simulink model "gtrackpol15"  (R2017a)
settings: Solver=ode45  StartTime=0.0  StopTime=15  FixedStep=.1  RelTol=1e-3
libraries: simulink x2
settings Model: Creator=Dell  LastModifiedBy=Dell
settings OptimizationCC: LifeSpan=inf
settings DebuggingCC: SFExecutionAtInitializationDiag=none
settings HardwareCC: ProdBitPerSizeT=32  ProdBitPerPtrDiffT=32  ProdWordSize=32  ProdHWDeviceType=Specified

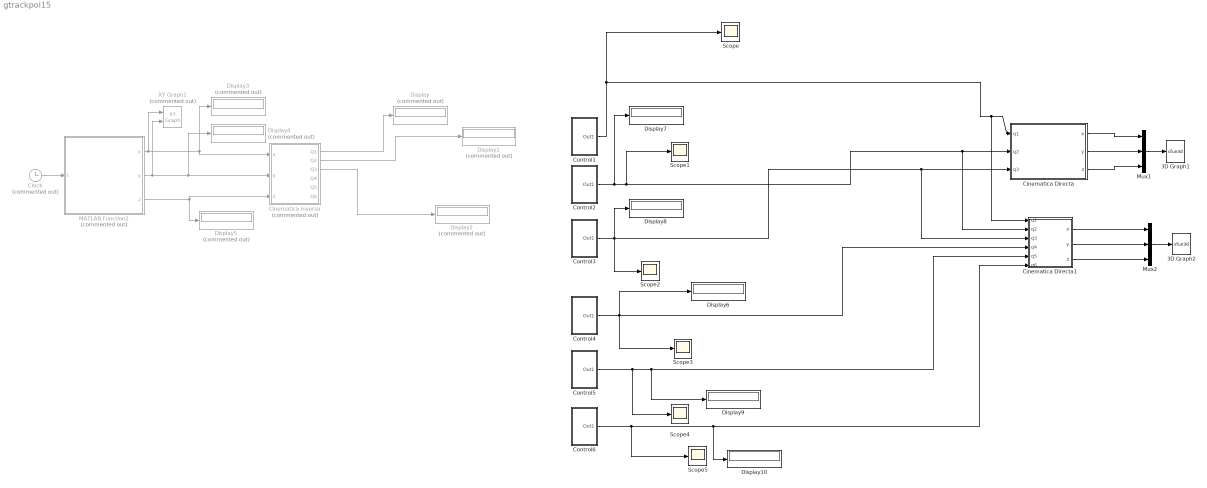
== system gtrackpol15 ==
  3D Graph1 : S-Function  LoadFcn=if exist('sfun3d','file'), sfun3d([],[],[],'LoadBlock'); end  FunctionName=sfun3d  Parameters=ax,T,np,cp,gd,ls,mk,mx,hd,tb  SFunctionDeploymentMode=off  EnableBusSupport=off  mask(3D Graph){np=1, ax=[-.7 0.7 -.7 0.7 -.7 .7], mx=2000, T=-1, cp=[370 -234 -207], gd=on, hd=on, tb=off, ls=-, mk=none}
      mask prompts: np "Number of moving points (lines)"; ax "Range: [xmin xmax  ymin ymax zmin zmax]"; mx "Max number of points in each line"; T "Sampling Time"; cp "Camera position (use [0 0 1] for 2D XY view)"; gd "Grid (on|off)"; hd "HeadMarkers (on|off)"; tb "Toolbar (on|off)"; ls "LineStyle"; mk "LineMarker"
      mask help:
      | This block plots the position of several points in the XYZ space. The input contains the coordinates of all the points (x1,y1,z1,x2,y2,z2,...).
      | The number of moving points (lines), the XYZ ranges, sampling time, camera position, and grid (among other things) can be set as mask parameters.
      settings: CopyFcn=if exist('sfun3d','file'), sfun3d([],[],[],'CopyBlock'); end  DeleteFcn=if exist('sfun3d','file'), sfun3d([],[],[],'DeleteBlock'); end  NameChangeFcn=if exist('sfun3d','file'), sfun3d([],[],[],'NameChange'); end
      mask Help:
      | This block plots the position of several points in the XYZ space. The input contains the coordinates of all the points (x1,y1,z1,x2,y2,z2,...).
      | The number of moving points (lines), the XYZ ranges, sampling time, camera position, and grid (among other things) can be set as mask parameters.
      mask TypeOptions ls: - | -- | : | -. | none
      mask TypeOptions mk: none | . | + | o | * | x | square | diamond | v | ^ | > | < | pentagram | hexagram
      mask Display: plot([.05 .95 .95 .05 .05],[.45 .45 .95 .95 .45], 0.5+cos(0:0.1:2*pi)*0.3,0.7+sin(0:0.1:2*pi)*0.2)
  3D Graph2 : S-Function  LoadFcn=if exist('sfun3d','file'), sfun3d([],[],[],'LoadBlock'); end  FunctionName=sfun3d  Parameters=ax,T,np,cp,gd,ls,mk,mx,hd,tb  SFunctionDeploymentMode=off  EnableBusSupport=off  mask(3D Graph){np=1, ax=[-.7 0.7 -.7 0.7 -.7 .7], mx=2000, T=-1, cp=[370 -234 -207], gd=on, hd=on, tb=off, ls=-, mk=none}
      mask prompts: np "Number of moving points (lines)"; ax "Range: [xmin xmax  ymin ymax zmin zmax]"; mx "Max number of points in each line"; T "Sampling Time"; cp "Camera position (use [0 0 1] for 2D XY view)"; gd "Grid (on|off)"; hd "HeadMarkers (on|off)"; tb "Toolbar (on|off)"; ls "LineStyle"; mk "LineMarker"
      mask help:
      | This block plots the position of several points in the XYZ space. The input contains the coordinates of all the points (x1,y1,z1,x2,y2,z2,...).
      | The number of moving points (lines), the XYZ ranges, sampling time, camera position, and grid (among other things) can be set as mask parameters.
      settings: CopyFcn=if exist('sfun3d','file'), sfun3d([],[],[],'CopyBlock'); end  DeleteFcn=if exist('sfun3d','file'), sfun3d([],[],[],'DeleteBlock'); end  NameChangeFcn=if exist('sfun3d','file'), sfun3d([],[],[],'NameChange'); end
      mask Help:
      | This block plots the position of several points in the XYZ space. The input contains the coordinates of all the points (x1,y1,z1,x2,y2,z2,...).
      | The number of moving points (lines), the XYZ ranges, sampling time, camera position, and grid (among other things) can be set as mask parameters.
      mask TypeOptions ls: - | -- | : | -. | none
      mask TypeOptions mk: none | . | + | o | * | x | square | diamond | v | ^ | > | < | pentagram | hexagram
      mask Display: plot([.05 .95 .95 .05 .05],[.45 .45 .95 .95 .45], 0.5+cos(0:0.1:2*pi)*0.3,0.7+sin(0:0.1:2*pi)*0.2)
  Cinematica Directa : MATLAB Function  TreatAsAtomicUnit=on
  Cinematica Directa1 : MATLAB Function  TreatAsAtomicUnit=on
  "Cinematica Inversa " : MATLAB Function  Commented=on  TreatAsAtomicUnit=on
  Clock : Clock  Commented=on
  "Control1 " : Subsystem
  Control2 : Subsystem
  "Control3 " : Subsystem
  "Control4 " : Subsystem
  Control5 : Subsystem
  Control6 : Subsystem
  Display{,1..5} (6 alike) : Display  Commented=on
  Display{6..10} (5 alike) : Display
  MATLAB Function2 : MATLAB Function  Commented=on  TreatAsAtomicUnit=on
  Mux1 : Mux  Inputs=3
  Mux2 : Mux  Inputs=3
  Scope{,1..5} (6 alike) : Scope
  XY Graph1 : simulink/Sinks/XY Graph  Commented=on  xmin=-1  xmax=1  ymin=-1  ymax=1  st=0.01
  wires:
  Control2/1(Out1) -> Cinematica Directa1/2(q2), Cinematica Directa/2(q2), Scope1/1, Display7/1
  MATLAB Function2/1(x) -> "Cinematica Inversa "/1(x), Display3/1, XY Graph1/1
  MATLAB Function2/3(z) -> "Cinematica Inversa "/3(z), Display5/1
  "Control1 "/1(Out1) -> Cinematica Directa1/1(q1), Cinematica Directa/1(q1), Scope/1
  "Cinematica Inversa "/3(Q3) -> Display2/1
  MATLAB Function2/2(y) -> XY Graph1/2, "Cinematica Inversa "/2(y), Display4/1
  "Cinematica Inversa "/2(Q2) -> Display1/1
  Clock/1 -> MATLAB Function2/1(t)
  "Cinematica Inversa "/1(Q1) -> Display/1
  Cinematica Directa/2(y) -> Mux1/2
  Cinematica Directa/3(z) -> Mux1/3
  Mux1/1 -> 3D Graph1/1
  Cinematica Directa/1(x) -> Mux1/1
  "Control3 "/1(Out1) -> Cinematica Directa1/3(q3), Cinematica Directa/3(q3), Scope2/1, Display8/1
  "Control4 "/1(Out1) -> Scope3/1, Display6/1, Cinematica Directa1/4(q4)
  Control5/1(Out1) -> Scope4/1, Display9/1, Cinematica Directa1/5(q5)
  Control6/1(Out1) -> Scope5/1, Display10/1, Cinematica Directa1/6(q6)
  Cinematica Directa1/1(x) -> Mux2/1
  Mux2/1 -> 3D Graph2/1
  Cinematica Directa1/3(z) -> Mux2/3
  Cinematica Directa1/2(y) -> Mux2/2

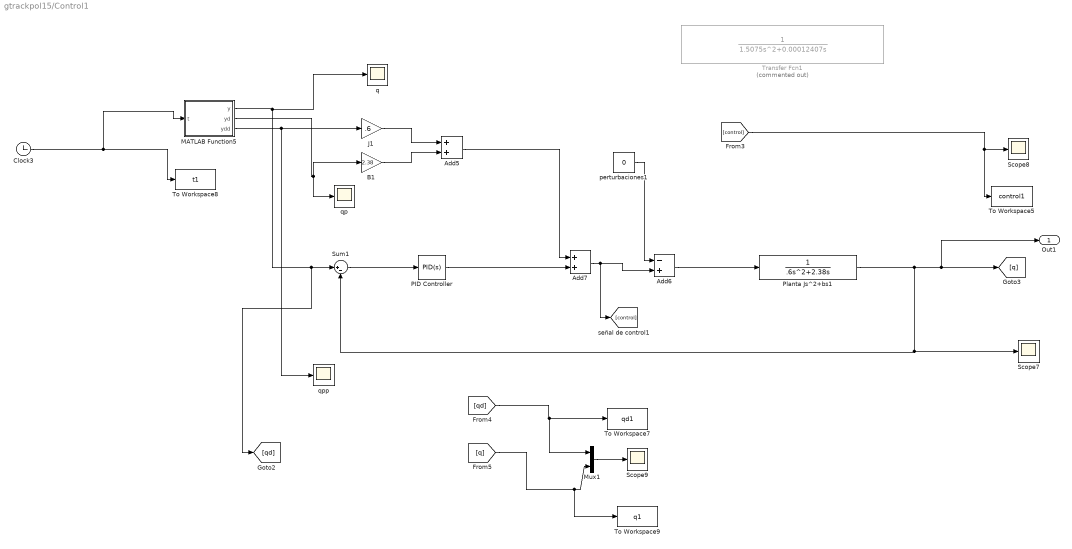
== system gtrackpol15/Control1  ==
  Add5 : Sum
  Add6 : Sum  Inputs=-+
  Add7 : Sum
  B1 : Gain  Gain=2.38
  Clock3 : Clock
  J1 : Gain  Gain=.6
  MATLAB Function5 : MATLAB Function  TreatAsAtomicUnit=on
  Mux1 : Mux  Inputs=2
  PID Controller : simulink/Continuous/PID Controller  Controller=PID  TimeDomain=Continuous-time  SampleTime=-1  IntegratorMethod=Forward Euler  FilterMethod=Forward Euler  Form=Parallel  UseFilter=on  ControllerParametersSource=internal  P=10  I=0  D=1  N=1279.60012976235  InitialConditionSource=internal  InitialConditionForIntegrator=0  InitialConditionForFilter=0  ExternalReset=none  LimitOutput=on  UpperSaturationLimit=255  LowerSaturationLimit=-255  LinearizeAsGain=on  AntiWindupMode=none  Kb=1  TrackingMode=off  Kt=1  PParamMin=[]  PParamMax=[]  IParamMin=[]  IParamMax=[]  DParamMin=[]  DParamMax=[]  NParamMin=[]  NParamMax=[]  KbParamMin=[]  KbParamMax=[]  KtParamMin=[]  KtParamMax=[]  POutMin=[]  POutMax=[]  IOutMin=[]  IOutMax=[]  DOutMin=[]  DOutMax=[]  NOutMin=[]  NOutMax=[]  KbOutMin=[]  KbOutMax=[]  KtOutMin=[]  KtOutMax=[]  IntegratorOutMin=[]  IntegratorOutMax=[]  FilterOutMin=[]  FilterOutMax=[]  SumOutMin=[]  SumOutMax=[]  SumI1OutMin=[]  SumI1OutMax=[]  SumI2OutMin=[]  SumI2OutMax=[]  SumI3OutMin=[]  SumI3OutMax=[]  SumDOutMin=[]  SumDOutMax=[]  SaturationOutMin=[]  SaturationOutMax=[]  IntegratorContinuousStateAttributes=''  IntegratorStateMustResolveToSignalObject=off  IntegratorRTWStateStorageClass=Auto  FilterContinuousStateAttributes=''  FilterStateMustResolveToSignalObject=off  FilterRTWStateStorageClass=Auto  DifferentiatorICPrevScaledInput=0  DifferentiatorOutMin=[]  DifferentiatorOutMax=[]  InitialConditionSetting=State (most efficient)
  Planta Js^2+bs1 : TransferFcn  Denominator=[.6 2.38 0]
  Scope7 : Scope
  Scope8 : Scope
  Scope9 : Scope
  Sum1 : Sum  Inputs=|+-
  To Workspace5 : ToWorkspace  VariableName=control1  SampleTime=-1
  To Workspace7 : ToWorkspace  VariableName=qd1  SampleTime=-1
  To Workspace8 : ToWorkspace  VariableName=t1  SampleTime=-1
  To Workspace9 : ToWorkspace  VariableName=q1  SampleTime=-1
  Transfer Fcn1 : TransferFcn  Commented=on  Denominator=[1.5075 0.00012407 0]
  perturbaciones1 : Constant  Value=0
  q : Scope
  qp : Scope
  qpp : Scope
  Out1 : Outport
  wires:
  MATLAB Function5/2(yd) -> B1/1, qp/1
  Mux1/1 -> Scope9/1
  Sum1/1 -> PID Controller/1
  J1/1 -> Add5/1
  Add7/1 -> Add6/2, [control]
  PID Controller/1 -> Add7/2
  [control] -> Scope8/1, To Workspace5/1
  [q] -> Mux1/2, To Workspace9/1
  [qd] -> Mux1/1, To Workspace7/1
  Add5/1 -> Add7/1
  Clock3/1 -> To Workspace8/1, MATLAB Function5/1(t)
  MATLAB Function5/1(y) -> q/1, Sum1/1, [qd]
  B1/1 -> Add5/2
  perturbaciones1/1 -> Add6/1
  MATLAB Function5/3(ydd) -> qpp/1, J1/1
  Add6/1 -> Planta Js^2+bs1/1
  Planta Js^2+bs1/1 -> Sum1/2, Scope7/1, Out1/1, [q]

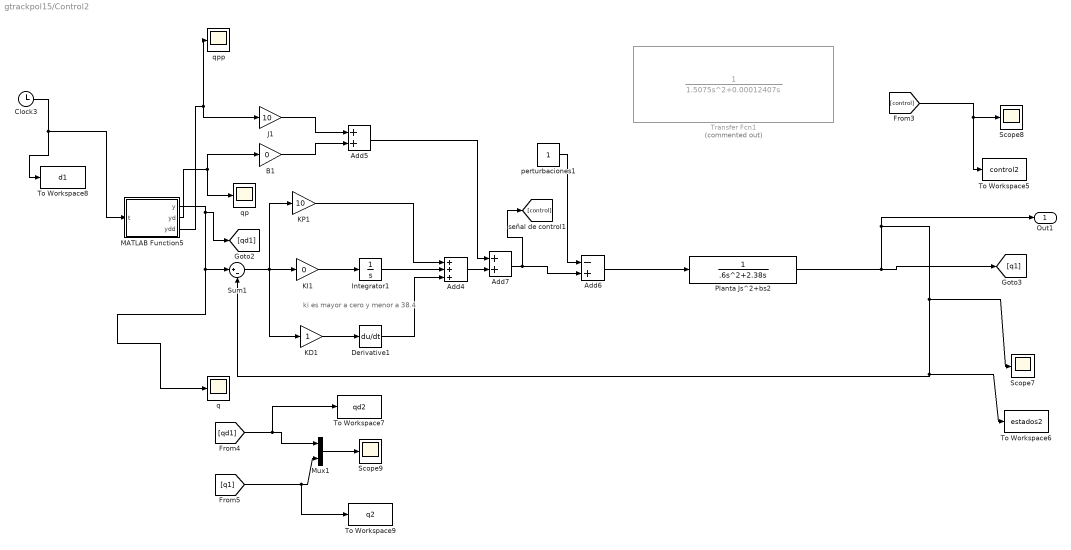
== system gtrackpol15/Control2 ==
  note: ki es mayor a cero y menor a 38.4
  Add4 : Sum  Inputs=+++
  Add5 : Sum
  Add6 : Sum  Inputs=-+
  Add7 : Sum
  B1 : Gain  Gain=0
  Clock3 : Clock
  Derivative1 : Derivative
  Integrator1 : Integrator
  J1 : Gain  Gain=10
  KD1 : Gain
  KI1 : Gain  Gain=0
  KP1 : Gain  Gain=10
  MATLAB Function5 : MATLAB Function  TreatAsAtomicUnit=on
  Mux1 : Mux  Inputs=2
  Planta Js^2+bs2 : TransferFcn  Denominator=[.6 2.38 0]
  Scope7 : Scope
  Scope8 : Scope
  Scope9 : Scope
  Sum1 : Sum  Inputs=|+-
  To Workspace5 : ToWorkspace  VariableName=control2  SampleTime=-1
  To Workspace6 : ToWorkspace  VariableName=estados2  SampleTime=-1
  To Workspace7 : ToWorkspace  VariableName=qd2  SampleTime=-1
  To Workspace8 : ToWorkspace  VariableName=d1  SampleTime=-1
  To Workspace9 : ToWorkspace  VariableName=q2  SampleTime=-1
  Transfer Fcn1 : TransferFcn  Commented=on  Denominator=[1.5075 0.00012407 0]
  perturbaciones1 : Constant
  q : Scope
  qp : Scope
  qpp : Scope
  Out1 : Outport
  wires:
  Derivative1/1 -> Add4/3
  perturbaciones1/1 -> Add6/1
  B1/1 -> Add5/2
  MATLAB Function5/1(y) -> [qd1], q/1, Sum1/1
  KD1/1 -> Derivative1/1
  Add5/1 -> Add7/1
  Integrator1/1 -> Add4/2
  MATLAB Function5/3(ydd) -> qpp/1, J1/1
  [qd1] -> To Workspace7/1, Mux1/1
  [q1] -> To Workspace9/1, Mux1/2
  KI1/1 -> Integrator1/1
  [control] -> To Workspace5/1, Scope8/1
  Add4/1 -> Add7/2
  Add7/1 -> [control], Add6/2
  J1/1 -> Add5/1
  Sum1/1 -> KD1/1, KI1/1, KP1/1
  Mux1/1 -> Scope9/1
  KP1/1 -> Add4/1
  MATLAB Function5/2(yd) -> qp/1, B1/1
  Add6/1 -> Planta Js^2+bs2/1
  Planta Js^2+bs2/1 -> Scope7/1, To Workspace6/1, Sum1/2, Out1/1, [q1]
  Clock3/1 -> MATLAB Function5/1(t), To Workspace8/1

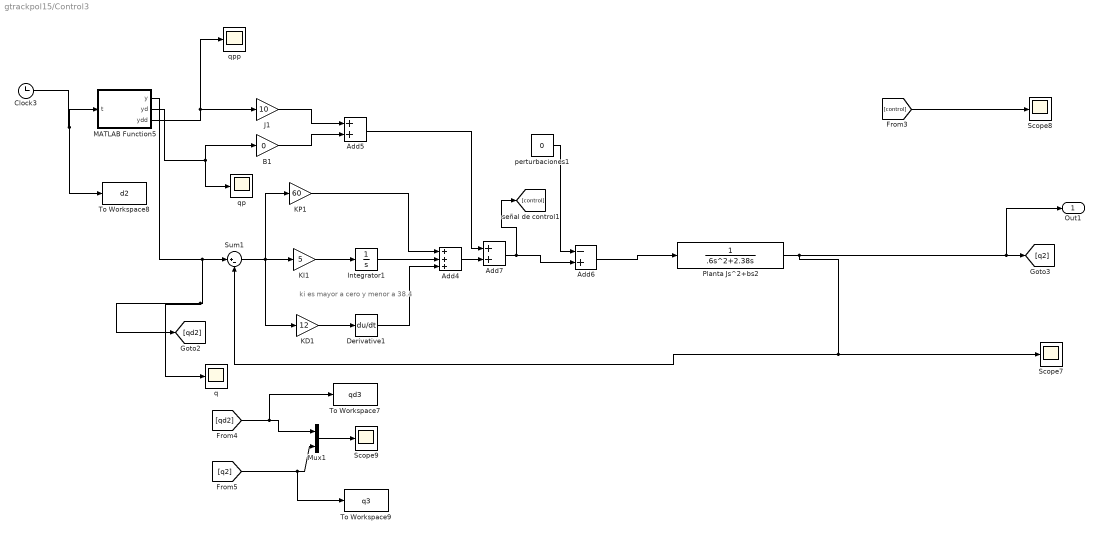
== system gtrackpol15/Control3  ==
  note: ki es mayor a cero y menor a 38.4
  Add4 : Sum  Inputs=+++
  Add5 : Sum
  Add6 : Sum  Inputs=-+
  Add7 : Sum
  B1 : Gain  Gain=0
  Clock3 : Clock
  Derivative1 : Derivative
  Integrator1 : Integrator
  J1 : Gain  Gain=10
  KD1 : Gain  Gain=12
  KI1 : Gain  Gain=5
  KP1 : Gain  Gain=60
  MATLAB Function5 : MATLAB Function  TreatAsAtomicUnit=on
  Mux1 : Mux  Inputs=2
  Planta Js^2+bs2 : TransferFcn  Denominator=[.6 2.38 0]
  Scope7 : Scope
  Scope8 : Scope
  Scope9 : Scope
  Sum1 : Sum  Inputs=|+-
  To Workspace7 : ToWorkspace  VariableName=qd3  SampleTime=-1
  To Workspace8 : ToWorkspace  VariableName=d2  SampleTime=-1
  To Workspace9 : ToWorkspace  VariableName=q3  SampleTime=-1
  perturbaciones1 : Constant  Value=0
  q : Scope
  qp : Scope
  qpp : Scope
  Out1 : Outport
  wires:
  MATLAB Function5/2(yd) -> B1/1, qp/1
  KP1/1 -> Add4/1
  Mux1/1 -> Scope9/1
  Sum1/1 -> KP1/1, KI1/1, KD1/1
  Planta Js^2+bs2/1 -> Sum1/2, Scope7/1, [q2], Out1/1
  J1/1 -> Add5/1
  Add7/1 -> Add6/2, [control]
  Add4/1 -> Add7/2
  [control] -> Scope8/1
  KI1/1 -> Integrator1/1
  [q2] -> Mux1/2, To Workspace9/1
  [qd2] -> Mux1/1, To Workspace7/1
  MATLAB Function5/3(ydd) -> qpp/1, J1/1
  Add6/1 -> Planta Js^2+bs2/1
  Integrator1/1 -> Add4/2
  Add5/1 -> Add7/1
  KD1/1 -> Derivative1/1
  MATLAB Function5/1(y) -> Sum1/1, [qd2], q/1
  B1/1 -> Add5/2
  perturbaciones1/1 -> Add6/1
  Derivative1/1 -> Add4/3
  Clock3/1 -> MATLAB Function5/1(t), To Workspace8/1

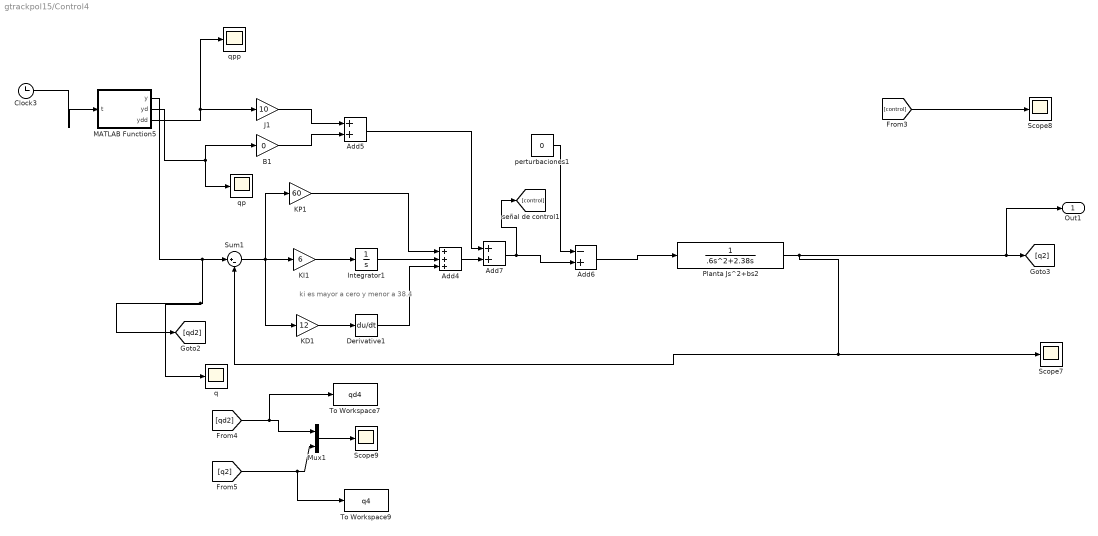
== system gtrackpol15/Control4  ==
  note: ki es mayor a cero y menor a 38.4
  Add4 : Sum  Inputs=+++
  Add5 : Sum
  Add6 : Sum  Inputs=-+
  Add7 : Sum
  B1 : Gain  Gain=0
  Clock3 : Clock
  Derivative1 : Derivative
  Integrator1 : Integrator
  J1 : Gain  Gain=10
  KD1 : Gain  Gain=12
  KI1 : Gain  Gain=6
  KP1 : Gain  Gain=60
  MATLAB Function5 : MATLAB Function  TreatAsAtomicUnit=on
  Mux1 : Mux  Inputs=2
  Planta Js^2+bs2 : TransferFcn  Denominator=[.6 2.38 0]
  Scope7 : Scope
  Scope8 : Scope
  Scope9 : Scope
  Sum1 : Sum  Inputs=|+-
  To Workspace7 : ToWorkspace  VariableName=qd4  SampleTime=-1
  To Workspace9 : ToWorkspace  VariableName=q4  SampleTime=-1
  perturbaciones1 : Constant  Value=0
  q : Scope
  qp : Scope
  qpp : Scope
  Out1 : Outport
  wires:
  MATLAB Function5/2(yd) -> B1/1, qp/1
  KP1/1 -> Add4/1
  Mux1/1 -> Scope9/1
  Sum1/1 -> KP1/1, KI1/1, KD1/1
  Planta Js^2+bs2/1 -> Sum1/2, Scope7/1, [q2], Out1/1
  J1/1 -> Add5/1
  Add7/1 -> Add6/2, [control]
  Add4/1 -> Add7/2
  [control] -> Scope8/1
  KI1/1 -> Integrator1/1
  [q2] -> Mux1/2, To Workspace9/1
  [qd2] -> Mux1/1, To Workspace7/1
  MATLAB Function5/3(ydd) -> qpp/1, J1/1
  Add6/1 -> Planta Js^2+bs2/1
  Integrator1/1 -> Add4/2
  Add5/1 -> Add7/1
  KD1/1 -> Derivative1/1
  MATLAB Function5/1(y) -> Sum1/1, [qd2], q/1
  B1/1 -> Add5/2
  perturbaciones1/1 -> Add6/1
  Derivative1/1 -> Add4/3
  Clock3/1 -> MATLAB Function5/1(t)

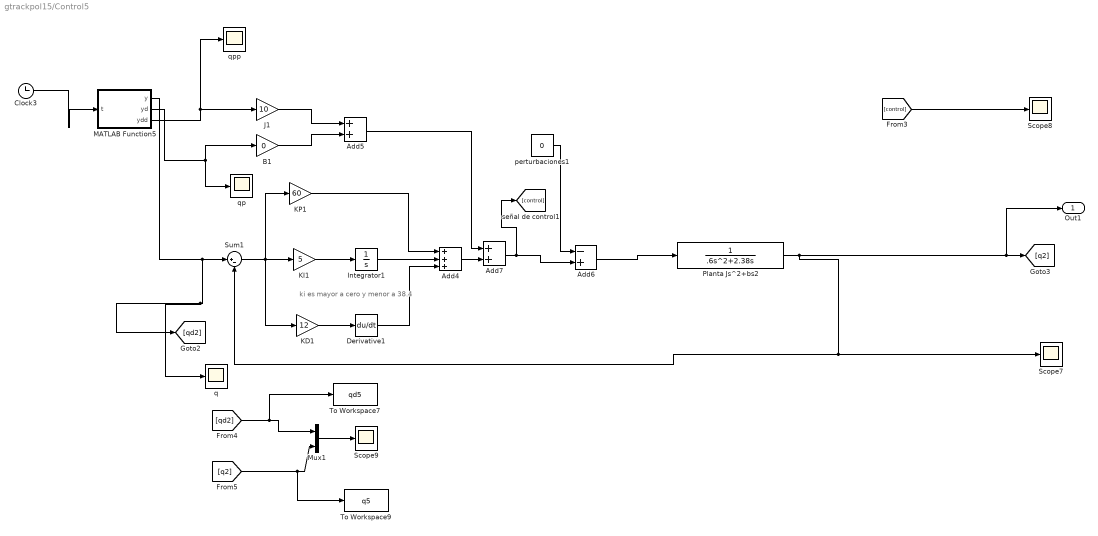
== system gtrackpol15/Control5 ==
  note: ki es mayor a cero y menor a 38.4
  Add4 : Sum  Inputs=+++
  Add5 : Sum
  Add6 : Sum  Inputs=-+
  Add7 : Sum
  B1 : Gain  Gain=0
  Clock3 : Clock
  Derivative1 : Derivative
  Integrator1 : Integrator
  J1 : Gain  Gain=10
  KD1 : Gain  Gain=12
  KI1 : Gain  Gain=5
  KP1 : Gain  Gain=60
  MATLAB Function5 : MATLAB Function  TreatAsAtomicUnit=on
  Mux1 : Mux  Inputs=2
  Planta Js^2+bs2 : TransferFcn  Denominator=[.6 2.38 0]
  Scope7 : Scope
  Scope8 : Scope
  Scope9 : Scope
  Sum1 : Sum  Inputs=|+-
  To Workspace7 : ToWorkspace  VariableName=qd5  SampleTime=-1
  To Workspace9 : ToWorkspace  VariableName=q5  SampleTime=-1
  perturbaciones1 : Constant  Value=0
  q : Scope
  qp : Scope
  qpp : Scope
  Out1 : Outport
  wires:
  MATLAB Function5/2(yd) -> B1/1, qp/1
  KP1/1 -> Add4/1
  Mux1/1 -> Scope9/1
  Sum1/1 -> KP1/1, KI1/1, KD1/1
  Planta Js^2+bs2/1 -> Sum1/2, Scope7/1, [q2], Out1/1
  J1/1 -> Add5/1
  Add7/1 -> Add6/2, [control]
  Add4/1 -> Add7/2
  [control] -> Scope8/1
  KI1/1 -> Integrator1/1
  [q2] -> Mux1/2, To Workspace9/1
  [qd2] -> Mux1/1, To Workspace7/1
  MATLAB Function5/3(ydd) -> qpp/1, J1/1
  Add6/1 -> Planta Js^2+bs2/1
  Integrator1/1 -> Add4/2
  Add5/1 -> Add7/1
  KD1/1 -> Derivative1/1
  MATLAB Function5/1(y) -> Sum1/1, [qd2], q/1
  B1/1 -> Add5/2
  perturbaciones1/1 -> Add6/1
  Derivative1/1 -> Add4/3
  Clock3/1 -> MATLAB Function5/1(t)

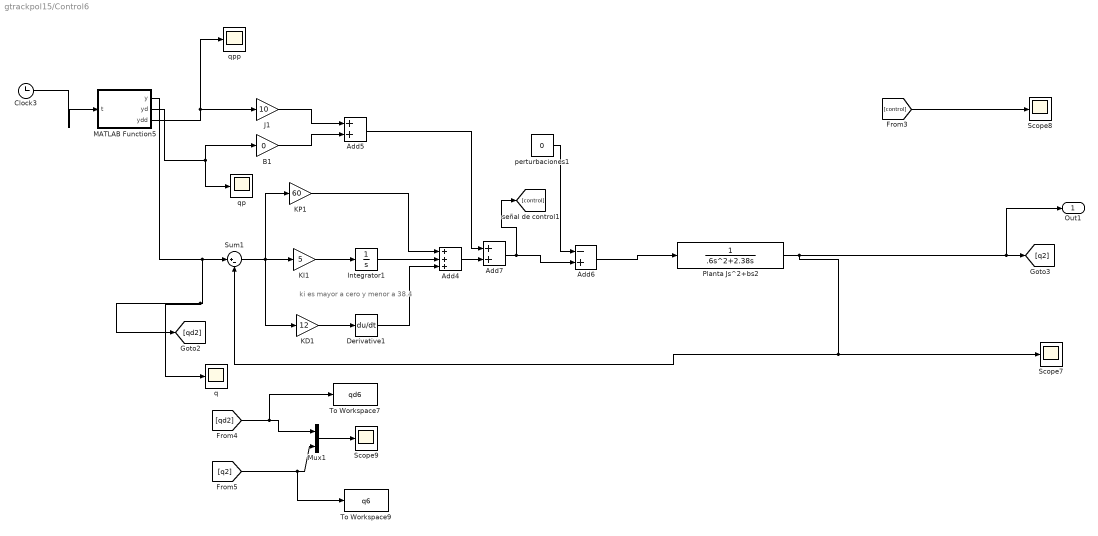
== system gtrackpol15/Control6 ==
  note: ki es mayor a cero y menor a 38.4
  Add4 : Sum  Inputs=+++
  Add5 : Sum
  Add6 : Sum  Inputs=-+
  Add7 : Sum
  B1 : Gain  Gain=0
  Clock3 : Clock
  Derivative1 : Derivative
  Integrator1 : Integrator
  J1 : Gain  Gain=10
  KD1 : Gain  Gain=12
  KI1 : Gain  Gain=5
  KP1 : Gain  Gain=60
  MATLAB Function5 : MATLAB Function  TreatAsAtomicUnit=on
  Mux1 : Mux  Inputs=2
  Planta Js^2+bs2 : TransferFcn  Denominator=[.6 2.38 0]
  Scope7 : Scope
  Scope8 : Scope
  Scope9 : Scope
  Sum1 : Sum  Inputs=|+-
  To Workspace7 : ToWorkspace  VariableName=qd6  SampleTime=-1
  To Workspace9 : ToWorkspace  VariableName=q6  SampleTime=-1
  perturbaciones1 : Constant  Value=0
  q : Scope
  qp : Scope
  qpp : Scope
  Out1 : Outport
  wires:
  MATLAB Function5/2(yd) -> B1/1, qp/1
  KP1/1 -> Add4/1
  Mux1/1 -> Scope9/1
  Sum1/1 -> KP1/1, KI1/1, KD1/1
  Planta Js^2+bs2/1 -> Sum1/2, Scope7/1, [q2], Out1/1
  J1/1 -> Add5/1
  Add7/1 -> Add6/2, [control]
  Add4/1 -> Add7/2
  [control] -> Scope8/1
  KI1/1 -> Integrator1/1
  [q2] -> Mux1/2, To Workspace9/1
  [qd2] -> Mux1/1, To Workspace7/1
  MATLAB Function5/3(ydd) -> qpp/1, J1/1
  Add6/1 -> Planta Js^2+bs2/1
  Integrator1/1 -> Add4/2
  Add5/1 -> Add7/1
  KD1/1 -> Derivative1/1
  MATLAB Function5/1(y) -> Sum1/1, [qd2], q/1
  B1/1 -> Add5/2
  perturbaciones1/1 -> Add6/1
  Derivative1/1 -> Add4/3
  Clock3/1 -> MATLAB Function5/1(t)

== matlab function gtrackpol15/Cinematica Directa ==
  data: x output; q1 input; y output; z output; q2 input; q3 input
function [x,y,z]= fcn(q1,q2,q3)
 %segunda CD es de alex                                                                                          
% longitud en metros 
l1=0.1794;
l2=.08490;
l3=0.12580;
l4=0.16579+.083;
l5=0.03;

%de 0 a 6 
% Pos=[l2*cos(q1) + l3*cos(q1)*cos(q2) + l4*cos(q1)*cos(q2)*cos(q3) - l4*cos(q1)*sin(q2)*sin(q3) + l5*sin(q1)*sin(q4)*sin(q5) + l5*cos(q1)*cos(q2)*cos(q3)*cos(q5) - l5*cos(q1)*cos(q5)*sin(q2)*sin(q3) - l5*cos(q1)*cos(q2)*cos(q4)*sin(q3)*sin(q5) - l5*cos(q1)*cos(q3)*cos(q4)*sin(q2)*sin(q5);
%     l2*sin(q1) + l3*cos(q2)*sin(q1) + l4*cos(q2)*cos(q3)*sin(q1) - l5*cos(q1)*sin(q4)*sin(q5) - l4*sin(q1)*sin(q2)*sin(q3) + l5*cos(q2)*cos(q3)*cos(q5)*sin(q1) - l5*cos(q5)*sin(q1)*sin(q2)*sin(q3) - l5*cos(q2)*cos(q4)*sin(q1)*sin(q3)*sin(q5) - l5*cos(q3)*cos(q4)*sin(q1)*sin(q2)*sin(q5); 
%     l1 + l3*sin(q2) + l4*cos(q2)*sin(q3) + l4*cos(q3)*sin(q2) + l5*cos(q2)*cos(q5)*sin(q3) + l5*cos(q3)*cos(q5)*sin(q2) + l5*cos(q2)*cos(q3)*cos(q4)*sin(q5) - l5*cos(q4)*sin(q2)*sin(q3)*sin(q5)]

%cinemática directa 
%x = Pos(1);
%y = Pos(2); %signo (- )para que cambie el cuadrante 
%z = Pos(3);


Pos=[cos(q1)*(l2 + l4*cos(q2 + q3) + l3*cos(q2));sin(q1)*(l2 + l4*cos(q2 + q3) + l3*cos(q2)); l1 + l4*sin(q2 + q3) + l3*sin(q2)];



x=Pos(1);
y=Pos(2);
z=Pos(3);

== matlab function gtrackpol15/Control2/MATLAB Function5 ==
  data: y output; t input; yd output; ydd output

function [y,yd,ydd] = qdd(t)
y=0;
yd=0;
ydd=0;
%a=[0 0 0 0 0 0]
if (t>0)&&(t<=3)
 
t0=0; tf=3; 
 v0=0; alpha0=0; qf=1.44 ; 
 vf=0; alphaf=0; q0=0;  
%vf alphaf q0 para efectos practicos



T=[1 t0  t0^2  t0^3   t0^4      t0^5;
   0  1 2*t0 3*t0^2 4*t0^3    5*t0^4;
   0  0   2   6*t0  12*t0^2   20*t0^3;
   1  tf  tf^2 tf^3  tf^4      tf^5;
   0  1   2*tf  3*tf^2  4*tf^3  5*tf^4;
   0  0   2      6*tf    12*tf^2  20*tf^3];  % le cambie l cubo en la terecera


g=[q0;v0;alpha0;qf;vf;alphaf];
a= T\g;    % a(1)= pos a(2)= vel   a(3)= acel
%primer punt0 

y= a(1)+a(2)*(t)+a(3)*(t.^2)+a(4)*(t.^3)+a(5)*(t.^4)+a(6)*(t.^5);
yd= a(2)+2*a(3)*(t)+3*a(4)*(t.^2)+4*a(5)*(t.^3)+5*a(6)*(t.^4);
ydd= 2*a(3)+6*a(4)*(t)+12*a(5)*(t.^2)+20*a(6)*(t.^3);

else
if (t>3)&&(t<=6)
    
    %% segundo punto 

t0=3; tf=6 
v0=0;  vf=0;
alpha0=0;  alphaf=0; 
q0=1.44; qf=1.1338; 



T=[1 t0  t0^2  t0^3   t0^4      t0^5;
   0  1 2*t0 3*t0^2 4*t0^3    5*t0^4;
   0  0   2   6*t0  12*t0^2   20*t0^3;
   1  tf  tf^2 tf^3  tf^4      tf^5;
   0  1   2*tf  3*tf^2  4*tf^3  5*tf^4;
   0  0   2      6*tf    12*tf^2  20*tf^3];


g=[q0;v0;alpha0;qf;vf;alphaf];
a=T\g;    % a(1)= pos a(2)= vel   a(3)= acel

y= a(1)+a(2)*(t)+a(3)*(t.^2)+a(4)*(t.^3)+a(5)*(t.^4)+a(6)*(t.^5);
yd= a(2)+2*a(3)*(t)+3*a(4)*(t.^2)+4*a(5)*(t.^3)+5*a(6)*(t.^4);
ydd= 2*a(3)+6*a(4)*(t)+12*a(5)*(t.^2)+20*a(6)*(t.^3);

else
 if (t>6)&&(t<=9)
%% tercer punto 
t0=6; tf=9;  
v0=0;  vf=0;
alpha0=0;   alphaf=0;
q0=1.1338; qf=1.1176;   

%vf alphaf q0 para efectos practicos


T=[1 t0  t0^2  t0^3   t0^4      t0^5;
   0  1 2*t0 3*t0^2 4*t0^3    5*t0^4;
   0  0   2   6*t0  12*t0^2   20*t0^3;
   1  tf  tf^2 tf^3  tf^4      tf^5;
   0  1   2*tf  3*tf^2  4*tf^3  5*tf^4;
   0  0   2      6*tf    12*tf^2  20*tf^3];

g=[q0;v0;alpha0;qf;vf;alphaf];
a=T\g;    % a(1)= pos a(2)= vel   a(3)= acel
%primer puntp q=[0 10] donde q=[q0 qf]
y= a(1)+a(2)*(t)+a(3)*(t.^2)+a(4)*(t.^3)+a(5)*(t.^4)+a(6)*(t.^5);
yd= a(2)+2*a(3)*(t)+3*a(4)*(t.^2)+4*a(5)*(t.^3)+5*a(6)*(t.^4);
ydd= 2*a(3)+6*a(4)*(t)+12*a(5)*(t.^2)+20*a(6)*(t.^3);

else
 if (t>9)&&(t<=12)
%% cuarto punto 
t0=9; tf=12;  v0=0; alpha0=0;   alphaf=0;  vf=0;  
q0=1.1176; qf=1.1039 ;

T=[1 t0  t0^2  t0^3   t0^4      t0^5;
   0  1 2*t0 3*t0^2 4*t0^3    5*t0^4;
   0  0   2   6*t0  12*t0^2   20*t0^3;
   1  tf  tf^2 tf^3  tf^4      tf^5;
   0  1   2*tf  3*tf^2  4*tf^3  5*tf^4;
   0  0   2      6*tf    12*tf^2  20*tf^3];


g=[q0;v0;alpha0;qf;vf;alphaf];
a=T\g;    % a(1)= pos a(2)= vel   a(3)= acel
%primer puntp q=[0 10] donde q=[q0 qf]

y= a(1)+a(2)*(t)+a(3)*(t.^2)+a(4)*(t.^3)+a(5)*(t.^4)+a(6)*(t.^5);
yd= a(2)+2*a(3)*(t)+3*a(4)*(t.^2)+4*a(5)*(t.^3)+5*a(6)*(t.^4);
ydd= 2*a(3)+6*a(4)*(t)+12*a(5)*(t.^2)+20*a(6)*(t.^3);

else
 if (t>12)&&(t<=15)
%% Quinto punto 
     t0=12; tf=15;  v0=0; alpha0=0; qf=1.099 ; alphaf=0; q0=1.1039; vf=0;  


T=[1 t0  t0^2  t0^3   t0^4      t0^5;
   0  1 2*t0 3*t0^2 4*t0^3    5*t0^4;
   0  0   2   6*t0  12*t0^2   20*t0^3;
   1  tf  tf^2 tf^3  tf^4      tf^5;
   0  1   2*tf  3*tf^2  4*tf^3  5*tf^4;
   0  0   2      6*tf    12*tf^2  20*tf^3];

g=[q0;v0;alpha0;qf;vf;alphaf];
a=T\g;    % a(1)= pos a(2)= vel   a(3)= acel

y= a(1)+a(2)*(t)+a(3)*(t.^2)+a(4)*(t.^3)+a(5)*(t.^4)+a(6)*(t.^5);
yd= a(2)+2*a(3)*(t)+3*a(4)*(t.^2)+4*a(5)*(t.^3)+5*a(6)*(t.^4);
ydd= 2*a(3)+6*a(4)*(t)+12*a(5)*(t.^2)+20*a(6)*(t.^3);

else
      if t>15
           ydd=0;
           yd=0;
           y=1.1;
      end
end
end
end
end
end

== matlab function gtrackpol15/MATLAB Function2 ==
  data: x output; t input; y output; z output
% function [x,y,z]= Trayectoria(t)
% x_c=0.1; %% x_c y y_c representa el centro
% y_c=0.15;
% r=0.05+0.08*sin(t); %% este es el radio de la figura
% x=x_c+r*sin(t);
% y=y_c+r*cos(t);
% z = 0.01;
% end 

%% Trayectoria para los polinomios
function [x,y,z] = fcn(t)
x=0;
y=0;
z=0;
if t>=0 && t<20
x=0.06;
y=0.078;
z=0.08;

elseif t>=20 && t<40
x=0.075;
y=0.080;
z=0.08;

elseif t>=40 && t<60
x=0.080;
y=0.085;
z=0.08;

elseif t>=60 && t<80
x=0.0350;
y=0.050;
z=0.08;

end

== matlab function gtrackpol15/Cinematica Inversa  ==
  data: Q1 output; x input; Q2 output; Q3 output; y input; z input; Q4 output; Q5 output; Q6 output
function [Q1,Q2,Q3,Q4,Q5,Q6] = fcn(x,y,z)
l1=0.1794;
l2=0.08490;
l3=0.12580;
l4=0.16579+.083;
l5=0.03;


%%%codo Arriba
r=sqrt(x^2+y^2);
ca=r-l2; %%
co=z-l1; %%
Q1 = atan2(y,x);
hi=sqrt(ca^2+co^2);
C3 =((-hi^2+l3^2+l4^2)/(-2*l4*l3));
Q3= atan2(sqrt(1-C3^2),C3); %%Codo Arriba
Q2=atan2(co,ca)-atan2(l4*sin(Q3),l3+l4*cos(Q3));


Q4=atan2(cos(Q1),sin(Q2+Q3)*sin(Q1))
Q5=atan2(-sqrt(1-(cos(Q2+Q3)*cos(Q1))),cos(Q2+Q3)*cos(Q1))
Q6=atan2(sin(Q2+Q3),cos(Q2+Q3)*cos(Q1))

== matlab function gtrackpol15/Control3 /MATLAB Function5 ==
  data: y output; t input; yd output; ydd output

function [y,yd,ydd] = qdd(t)
y=0;
yd=0;
ydd=0;
%a=[0 0 0 0 0 0]
if (t>0)&&(t<=3)
 
t0=0; tf=3; 
 v0=0; alpha0=0; qf=-2.69 ; 
 vf=0; alphaf=0; q0=0;  
%vf alphaf q0 para efectos practicos



T=[1 t0  t0^2  t0^3   t0^4      t0^5;
   0  1 2*t0 3*t0^2 4*t0^3    5*t0^4;
   0  0   2   6*t0  12*t0^2   20*t0^3;
   1  tf  tf^2 tf^3  tf^4      tf^5;
   0  1   2*tf  3*tf^2  4*tf^3  5*tf^4;
   0  0   2      6*tf    12*tf^2  20*tf^3];  % le cambie l cubo en la terecera


g=[q0;v0;alpha0;qf;vf;alphaf];
a= T\g;    % a(1)= pos a(2)= vel   a(3)= acel
%primer punt0 

y= a(1)+a(2)*(t)+a(3)*(t.^2)+a(4)*(t.^3)+a(5)*(t.^4)+a(6)*(t.^5);
yd= a(2)+2*a(3)*(t)+3*a(4)*(t.^2)+4*a(5)*(t.^3)+5*a(6)*(t.^4);
ydd= 2*a(3)+6*a(4)*(t)+12*a(5)*(t.^2)+20*a(6)*(t.^3);

else
if (t>3)&&(t<=6)
    
    %% segundo punto 

t0=3; tf=6 
v0=0;  vf=0;
alpha0=0;  alphaf=0; 
q0=-2.69; qf=-2.6481; 



T=[1 t0  t0^2  t0^3   t0^4      t0^5;
   0  1 2*t0 3*t0^2 4*t0^3    5*t0^4;
   0  0   2   6*t0  12*t0^2   20*t0^3;
   1  tf  tf^2 tf^3  tf^4      tf^5;
   0  1   2*tf  3*tf^2  4*tf^3  5*tf^4;
   0  0   2      6*tf    12*tf^2  20*tf^3];


g=[q0;v0;alpha0;qf;vf;alphaf];
a=T\g;    % a(1)= pos a(2)= vel   a(3)= acel

y= a(1)+a(2)*(t)+a(3)*(t.^2)+a(4)*(t.^3)+a(5)*(t.^4)+a(6)*(t.^5);
yd= a(2)+2*a(3)*(t)+3*a(4)*(t.^2)+4*a(5)*(t.^3)+5*a(6)*(t.^4);
ydd= 2*a(3)+6*a(4)*(t)+12*a(5)*(t.^2)+20*a(6)*(t.^3);

else
 if (t>6)&&(t<=9)
%% tercer punto 
t0=6; tf=9;  
v0=0;  vf=0;
alpha0=0;   alphaf=0;
q0=-2.6481; qf=-2.58;   

%vf alphaf q0 para efectos practicos


T=[1 t0  t0^2  t0^3   t0^4      t0^5;
   0  1 2*t0 3*t0^2 4*t0^3    5*t0^4;
   0  0   2   6*t0  12*t0^2   20*t0^3;
   1  tf  tf^2 tf^3  tf^4      tf^5;
   0  1   2*tf  3*tf^2  4*tf^3  5*tf^4;
   0  0   2      6*tf    12*tf^2  20*tf^3];

g=[q0;v0;alpha0;qf;vf;alphaf];
a=T\g;    % a(1)= pos a(2)= vel   a(3)= acel
%primer puntp q=[0 10] donde q=[q0 qf]
y= a(1)+a(2)*(t)+a(3)*(t.^2)+a(4)*(t.^3)+a(5)*(t.^4)+a(6)*(t.^5);
yd= a(2)+2*a(3)*(t)+3*a(4)*(t.^2)+4*a(5)*(t.^3)+5*a(6)*(t.^4);
ydd= 2*a(3)+6*a(4)*(t)+12*a(5)*(t.^2)+20*a(6)*(t.^3);

else
 if (t>9)&&(t<=12)
%% cuarto punto 
t0=9; tf=12;  v0=0; alpha0=0;  alphaf=0;  vf=0;  
qf=-2.5498 ;  q0=-2.58;

T=[1 t0  t0^2  t0^3   t0^4      t0^5;
   0  1 2*t0 3*t0^2 4*t0^3    5*t0^4;
   0  0   2   6*t0  12*t0^2   20*t0^3;
   1  tf  tf^2 tf^3  tf^4      tf^5;
   0  1   2*tf  3*tf^2  4*tf^3  5*tf^4;
   0  0   2      6*tf    12*tf^2  20*tf^3];


g=[q0;v0;alpha0;qf;vf;alphaf];
a=T\g;    % a(1)= pos a(2)= vel   a(3)= acel
%primer puntp q=[0 10] donde q=[q0 qf]

y= a(1)+a(2)*(t)+a(3)*(t.^2)+a(4)*(t.^3)+a(5)*(t.^4)+a(6)*(t.^5);
yd= a(2)+2*a(3)*(t)+3*a(4)*(t.^2)+4*a(5)*(t.^3)+5*a(6)*(t.^4);
ydd= 2*a(3)+6*a(4)*(t)+12*a(5)*(t.^2)+20*a(6)*(t.^3);

 else  
 if (t>12)&&(t<=15)
%% Qinto punto 
     t0=12; tf=15;  v0=0; alpha0=0; qf=-2.80; alphaf=0; q0=-2.5498; vf=0;  


T=[1 t0  t0^2  t0^3   t0^4      t0^5;
   0  1 2*t0 3*t0^2 4*t0^3    5*t0^4;
   0  0   2   6*t0  12*t0^2   20*t0^3;
   1  tf  tf^2 tf^3  tf^4      tf^5;
   0  1   2*tf  3*tf^2  4*tf^3  5*tf^4;
   0  0   2      6*tf    12*tf^2  20*tf^3];

g=[q0;v0;alpha0;qf;vf;alphaf];
a=T\g;    % a(1)= pos a(2)= vel   a(3)= acel

y= a(1)+a(2)*(t)+a(3)*(t.^2)+a(4)*(t.^3)+a(5)*(t.^4)+a(6)*(t.^5);
yd= a(2)+2*a(3)*(t)+3*a(4)*(t.^2)+4*a(5)*(t.^3)+5*a(6)*(t.^4);
ydd= 2*a(3)+6*a(4)*(t)+12*a(5)*(t.^2)+20*a(6)*(t.^3);

else
      if t>15
           ydd=0;
           yd=0;
           y=0;
      end
end
end
end
end
end

== matlab function gtrackpol15/Cinematica Directa1 ==
  data: x output; q1 input; y output; z output; q2 input; q3 input; q4 input; q5 input; q6 input
function [x,y,z]= fcn(q1,q2,q3,q4,q5,q6)
 %segunda CD es de alex                                                                                          
% longitud en metros 
l1=0.1794;
l2=.08490;
l3=0.12580;
l4=0.16579+.083;
l5=0.03;
%%Pos= [l4*cos(q2)*cos(q3)*sin(q1) - l3*cos(q2)*sin(q1) - l2*sin(q1) + l5*cos(q1)*sin(q4)*sin(q5) - l4*sin(q1)*sin(q2)*sin(q3) + l5*cos(q2)*cos(q3)*cos(q5)*sin(q1) - l5*cos(q5)*sin(q1)*sin(q2)*sin(q3) - l5*cos(q2)*cos(q4)*sin(q1)*sin(q3)*sin(q5) - l5*cos(q3)*cos(q4)*sin(q1)*sin(q2)*sin(q5); l2*cos(q1) + l3*cos(q1)*cos(q2) - l4*cos(q1)*cos(q2)*cos(q3) + l4*cos(q1)*sin(q2)*sin(q3) + l5*sin(q1)*sin(q4)*sin(q5) - l5*cos(q1)*cos(q2)*cos(q3)*cos(q5) + l5*cos(q1)*cos(q5)*sin(q2)*sin(q3) + l5*cos(q1)*cos(q2)*cos(q4)*sin(q3)*sin(q5) + l5*cos(q1)*cos(q3)*cos(q4)*sin(q2)*sin(q5); l1 + l3*sin(q2) - l4*cos(q2)*sin(q3) - l4*cos(q3)*sin(q2) - l5*cos(q2)*cos(q5)*sin(q3) - l5*cos(q3)*cos(q5)*sin(q2) - l5*cos(q2)*cos(q3)*cos(q4)*sin(q5) + l5*cos(q4)*sin(q2)*sin(q3)*sin(q5)];
%%Pos=[-sin(q1)*(l2 - l4*cos(q2 + q3) + l3*cos(q2)); cos(q1)*(l2 - l4*cos(q2 + q3) + l3*cos(q2)); l1 - l4*sin(q2 + q3) + l3*sin(q2)]
%Pos=[cos(q1)*(l2 - l4*cos(q2 + q3) + l3*cos(q2)); 
%    sin(q1)*(l2 - l4*cos(q2 + q3) + l3*cos(q2)); 
%    l1 + l4*sin(q2 + q3) - l3*sin(q2)]
%%%Pos=[cos(q1)*(l2 + l4*cos(q2 + q3) + l3*cos(q2));
%%%    sin(q1)*(l2 + l4*cos(q2 + q3) + l3*cos(q2)); 
%%%    l1 + l4*sin(q2 + q3) + l3*sin(q2)]
Pos=[l2*cos(q1) + l3*cos(q1)*cos(q2) + l4*cos(q1)*cos(q2)*cos(q3) - l4*cos(q1)*sin(q2)*sin(q3) + l5*sin(q1)*sin(q4)*sin(q5) + l5*cos(q1)*cos(q2)*cos(q3)*cos(q5) - l5*cos(q1)*cos(q5)*sin(q2)*sin(q3) - l5*cos(q1)*cos(q2)*cos(q4)*sin(q3)*sin(q5) - l5*cos(q1)*cos(q3)*cos(q4)*sin(q2)*sin(q5);
    l2*sin(q1) + l3*cos(q2)*sin(q1) + l4*cos(q2)*cos(q3)*sin(q1) - l5*cos(q1)*sin(q4)*sin(q5) - l4*sin(q1)*sin(q2)*sin(q3) + l5*cos(q2)*cos(q3)*cos(q5)*sin(q1) - l5*cos(q5)*sin(q1)*sin(q2)*sin(q3) - l5*cos(q2)*cos(q4)*sin(q1)*sin(q3)*sin(q5) - l5*cos(q3)*cos(q4)*sin(q1)*sin(q2)*sin(q5); 
    l1 + l3*sin(q2) + l4*cos(q2)*sin(q3) + l4*cos(q3)*sin(q2) + l5*cos(q2)*cos(q5)*sin(q3) + l5*cos(q3)*cos(q5)*sin(q2) + l5*cos(q2)*cos(q3)*cos(q4)*sin(q5) - l5*cos(q4)*sin(q2)*sin(q3)*sin(q5)]

%cinemática directa 
%x = Pos(1);
%y = Pos(2); %signo (- )para que cambie el cuadrante 
%z = Pos(3);

x=Pos(1);
y=Pos(2);
z=Pos(3);

== matlab function gtrackpol15/Control4 /MATLAB Function5 ==
  data: y output; t input; yd output; ydd output

function [y,yd,ydd] = qdd(t)
y=0;
yd=0;
ydd=0;
%a=[0 0 0 0 0 0]
if (t>0)&&(t<=3)
 
t0=0; tf=3; 
 v0=0; alpha0=0; qf= 2.35 ; 
 vf=0; alphaf=0; q0=0;  
%vf alphaf q0 para efectos practicos



T=[1 t0  t0^2  t0^3   t0^4      t0^5;
   0  1 2*t0 3*t0^2 4*t0^3    5*t0^4;
   0  0   2   6*t0  12*t0^2   20*t0^3;
   1  tf  tf^2 tf^3  tf^4      tf^5;
   0  1   2*tf  3*tf^2  4*tf^3  5*tf^4;
   0  0   2      6*tf    12*tf^2  20*tf^3];  % le cambie l cubo en la terecera


g=[q0;v0;alpha0;qf;vf;alphaf];
a= T\g;    % a(1)= pos a(2)= vel   a(3)= acel
%primer punt0 

y= a(1)+a(2)*(t)+a(3)*(t.^2)+a(4)*(t.^3)+a(5)*(t.^4)+a(6)*(t.^5);
yd= a(2)+2*a(3)*(t)+3*a(4)*(t.^2)+4*a(5)*(t.^3)+5*a(6)*(t.^4);
ydd= 2*a(3)+6*a(4)*(t)+12*a(5)*(t.^2)+20*a(6)*(t.^3);

else
if (t>3)&&(t<=6)
    
    %% segundo punto 

t0=3; tf=6 
v0=0;  vf=0;
alpha0=0;  alphaf=0; 
q0=2.35; qf=2.485; 



T=[1 t0  t0^2  t0^3   t0^4      t0^5;
   0  1 2*t0 3*t0^2 4*t0^3    5*t0^4;
   0  0   2   6*t0  12*t0^2   20*t0^3;
   1  tf  tf^2 tf^3  tf^4      tf^5;
   0  1   2*tf  3*tf^2  4*tf^3  5*tf^4;
   0  0   2      6*tf    12*tf^2  20*tf^3];


g=[q0;v0;alpha0;qf;vf;alphaf];
a=T\g;    % a(1)= pos a(2)= vel   a(3)= acel

y= a(1)+a(2)*(t)+a(3)*(t.^2)+a(4)*(t.^3)+a(5)*(t.^4)+a(6)*(t.^5);
yd= a(2)+2*a(3)*(t)+3*a(4)*(t.^2)+4*a(5)*(t.^3)+5*a(6)*(t.^4);
ydd= 2*a(3)+6*a(4)*(t)+12*a(5)*(t.^2)+20*a(6)*(t.^3);

else
 if (t>6)&&(t<=9)
%% tercer punto 
t0=6; tf=9;  
v0=0;  vf=0;
alpha0=0;   alphaf=0;
q0=2.485; qf=2.38;   

%vf alphaf q0 para efectos practicos


T=[1 t0  t0^2  t0^3   t0^4      t0^5;
   0  1 2*t0 3*t0^2 4*t0^3    5*t0^4;
   0  0   2   6*t0  12*t0^2   20*t0^3;
   1  tf  tf^2 tf^3  tf^4      tf^5;
   0  1   2*tf  3*tf^2  4*tf^3  5*tf^4;
   0  0   2      6*tf    12*tf^2  20*tf^3];

g=[q0;v0;alpha0;qf;vf;alphaf];
a=T\g;    % a(1)= pos a(2)= vel   a(3)= acel
%primer puntp q=[0 10] donde q=[q0 qf]
y= a(1)+a(2)*(t)+a(3)*(t.^2)+a(4)*(t.^3)+a(5)*(t.^4)+a(6)*(t.^5);
yd= a(2)+2*a(3)*(t)+3*a(4)*(t.^2)+4*a(5)*(t.^3)+5*a(6)*(t.^4);
ydd= 2*a(3)+6*a(4)*(t)+12*a(5)*(t.^2)+20*a(6)*(t.^3);

else
 if (t>9)&&(t<=12)
%% cuarto punto 
t0=9; tf=12;  v0=0; alpha0=0; qf=2.3823 ;  alphaf=0; q0=2.38; vf=0;  


T=[1 t0  t0^2  t0^3   t0^4      t0^5;
   0  1 2*t0 3*t0^2 4*t0^3    5*t0^4;
   0  0   2   6*t0  12*t0^2   20*t0^3;
   1  tf  tf^2 tf^3  tf^4      tf^5;
   0  1   2*tf  3*tf^2  4*tf^3  5*tf^4;
   0  0   2      6*tf    12*tf^2  20*tf^3];


g=[q0;v0;alpha0;qf;vf;alphaf];
a=T\g;    % a(1)= pos a(2)= vel   a(3)= acel
%primer puntp q=[0 10] donde q=[q0 qf]

y= a(1)+a(2)*(t)+a(3)*(t.^2)+a(4)*(t.^3)+a(5)*(t.^4)+a(6)*(t.^5);
yd= a(2)+2*a(3)*(t)+3*a(4)*(t.^2)+4*a(5)*(t.^3)+5*a(6)*(t.^4);
ydd= 2*a(3)+6*a(4)*(t)+12*a(5)*(t.^2)+20*a(6)*(t.^3);

else
 if (t>12)&&(t<=15)

     t0=12; tf=15;  v0=0; alpha0=0; qf=2.52; alphaf=0; q0=2.3823; vf=0;  


T=[1 t0  t0^2  t0^3   t0^4      t0^5;
   0  1 2*t0 3*t0^2 4*t0^3    5*t0^4;
   0  0   2   6*t0  12*t0^2   20*t0^3;
   1  tf  tf^2 tf^3  tf^4      tf^5;
   0  1   2*tf  3*tf^2  4*tf^3  5*tf^4;
   0  0   2      6*tf    12*tf^2  20*tf^3];

g=[q0;v0;alpha0;qf;vf;alphaf];
a=T\g;    % a(1)= pos a(2)= vel   a(3)= acel

y= a(1)+a(2)*(t)+a(3)*(t.^2)+a(4)*(t.^3)+a(5)*(t.^4)+a(6)*(t.^5);
yd= a(2)+2*a(3)*(t)+3*a(4)*(t.^2)+4*a(5)*(t.^3)+5*a(6)*(t.^4);
ydd= 2*a(3)+6*a(4)*(t)+12*a(5)*(t.^2)+20*a(6)*(t.^3);

else
      if t>15
           ydd=0;
           yd=0;
           y=0;
      end
end
end
end
end
end

== matlab function gtrackpol15/Control5/MATLAB Function5 ==
  data: y output; t input; yd output; ydd output

function [y,yd,ydd] = qdd(t)
y=0;
yd=0;
ydd=0;
%a=[0 0 0 0 0 0]
if (t>0)&&(t<=3)
 
t0=0; tf=3; 
 v0=0; alpha0=0; qf=-2.69 ; 
 vf=0; alphaf=0; q0=0;  
%vf alphaf q0 para efectos practicos



T=[1 t0  t0^2  t0^3   t0^4      t0^5;
   0  1 2*t0 3*t0^2 4*t0^3    5*t0^4;
   0  0   2   6*t0  12*t0^2   20*t0^3;
   1  tf  tf^2 tf^3  tf^4      tf^5;
   0  1   2*tf  3*tf^2  4*tf^3  5*tf^4;
   0  0   2      6*tf    12*tf^2  20*tf^3];  % le cambie l cubo en la terecera


g=[q0;v0;alpha0;qf;vf;alphaf];
a= T\g;    % a(1)= pos a(2)= vel   a(3)= acel
%primer punt0 

y= a(1)+a(2)*(t)+a(3)*(t.^2)+a(4)*(t.^3)+a(5)*(t.^4)+a(6)*(t.^5);
yd= a(2)+2*a(3)*(t)+3*a(4)*(t.^2)+4*a(5)*(t.^3)+5*a(6)*(t.^4);
ydd= 2*a(3)+6*a(4)*(t)+12*a(5)*(t.^2)+20*a(6)*(t.^3);

else
if (t>3)&&(t<=6)
    
    %% segundo punto 

t0=3; tf=6 
v0=0;  vf=0;
alpha0=0;  alphaf=0; 
q0=-2.69; qf=-2.6481; 



T=[1 t0  t0^2  t0^3   t0^4      t0^5;
   0  1 2*t0 3*t0^2 4*t0^3    5*t0^4;
   0  0   2   6*t0  12*t0^2   20*t0^3;
   1  tf  tf^2 tf^3  tf^4      tf^5;
   0  1   2*tf  3*tf^2  4*tf^3  5*tf^4;
   0  0   2      6*tf    12*tf^2  20*tf^3];


g=[q0;v0;alpha0;qf;vf;alphaf];
a=T\g;    % a(1)= pos a(2)= vel   a(3)= acel

y= a(1)+a(2)*(t)+a(3)*(t.^2)+a(4)*(t.^3)+a(5)*(t.^4)+a(6)*(t.^5);
yd= a(2)+2*a(3)*(t)+3*a(4)*(t.^2)+4*a(5)*(t.^3)+5*a(6)*(t.^4);
ydd= 2*a(3)+6*a(4)*(t)+12*a(5)*(t.^2)+20*a(6)*(t.^3);

else
 if (t>6)&&(t<=9)
%% tercer punto 
t0=6; tf=9;  
v0=0;  vf=0;
alpha0=0;   alphaf=0;
q0=-2.6481; qf=-2.58;   

%vf alphaf q0 para efectos practicos


T=[1 t0  t0^2  t0^3   t0^4      t0^5;
   0  1 2*t0 3*t0^2 4*t0^3    5*t0^4;
   0  0   2   6*t0  12*t0^2   20*t0^3;
   1  tf  tf^2 tf^3  tf^4      tf^5;
   0  1   2*tf  3*tf^2  4*tf^3  5*tf^4;
   0  0   2      6*tf    12*tf^2  20*tf^3];

g=[q0;v0;alpha0;qf;vf;alphaf];
a=T\g;    % a(1)= pos a(2)= vel   a(3)= acel
%primer puntp q=[0 10] donde q=[q0 qf]
y= a(1)+a(2)*(t)+a(3)*(t.^2)+a(4)*(t.^3)+a(5)*(t.^4)+a(6)*(t.^5);
yd= a(2)+2*a(3)*(t)+3*a(4)*(t.^2)+4*a(5)*(t.^3)+5*a(6)*(t.^4);
ydd= 2*a(3)+6*a(4)*(t)+12*a(5)*(t.^2)+20*a(6)*(t.^3);

else
 if (t>9)&&(t<=12)
%% cuarto punto 
t0=9; tf=12;  v0=0; alpha0=0; qf=-2.5498 ;  alphaf=0; q0=-2.58; vf=0;  


T=[1 t0  t0^2  t0^3   t0^4      t0^5;
   0  1 2*t0 3*t0^2 4*t0^3    5*t0^4;
   0  0   2   6*t0  12*t0^2   20*t0^3;
   1  tf  tf^2 tf^3  tf^4      tf^5;
   0  1   2*tf  3*tf^2  4*tf^3  5*tf^4;
   0  0   2      6*tf    12*tf^2  20*tf^3];


g=[q0;v0;alpha0;qf;vf;alphaf];
a=T\g;    % a(1)= pos a(2)= vel   a(3)= acel
%primer puntp q=[0 10] donde q=[q0 qf]

y= a(1)+a(2)*(t)+a(3)*(t.^2)+a(4)*(t.^3)+a(5)*(t.^4)+a(6)*(t.^5);
yd= a(2)+2*a(3)*(t)+3*a(4)*(t.^2)+4*a(5)*(t.^3)+5*a(6)*(t.^4);
ydd= 2*a(3)+6*a(4)*(t)+12*a(5)*(t.^2)+20*a(6)*(t.^3);

else
 if (t>12)&&(t<=15)
 %% Quinto punto
     t0=12; tf=15;  v0=0; alpha0=0; qf=-2.80; alphaf=0; q0=-2.5498; vf=0;  


T=[1 t0  t0^2  t0^3   t0^4      t0^5;
   0  1 2*t0 3*t0^2 4*t0^3    5*t0^4;
   0  0   2   6*t0  12*t0^2   20*t0^3;
   1  tf  tf^2 tf^3  tf^4      tf^5;
   0  1   2*tf  3*tf^2  4*tf^3  5*tf^4;
   0  0   2      6*tf    12*tf^2  20*tf^3];

g=[q0;v0;alpha0;qf;vf;alphaf];
a=T\g;    % a(1)= pos a(2)= vel   a(3)= acel

y= a(1)+a(2)*(t)+a(3)*(t.^2)+a(4)*(t.^3)+a(5)*(t.^4)+a(6)*(t.^5);
yd= a(2)+2*a(3)*(t)+3*a(4)*(t.^2)+4*a(5)*(t.^3)+5*a(6)*(t.^4);
ydd= 2*a(3)+6*a(4)*(t)+12*a(5)*(t.^2)+20*a(6)*(t.^3);

else
      if t>15
           ydd=0;
           yd=0;
           y=0;
      end
end
end
end
end
end

== matlab function gtrackpol15/Control6/MATLAB Function5 ==
  data: y output; t input; yd output; ydd output

function [y,yd,ydd] = qdd(t)
y=0;
yd=0;
ydd=0;
%a=[0 0 0 0 0 0]
if (t>0)&&(t<=3)
 
t0=0; tf=3; 
 v0=0; alpha0=0; qf=-2.69 ; 
 vf=0; alphaf=0; q0=0;  
%vf alphaf q0 para efectos practicos



T=[1 t0  t0^2  t0^3   t0^4      t0^5;
   0  1 2*t0 3*t0^2 4*t0^3    5*t0^4;
   0  0   2   6*t0  12*t0^2   20*t0^3;
   1  tf  tf^2 tf^3  tf^4      tf^5;
   0  1   2*tf  3*tf^2  4*tf^3  5*tf^4;
   0  0   2      6*tf    12*tf^2  20*tf^3];  % le cambie l cubo en la terecera


g=[q0;v0;alpha0;qf;vf;alphaf];
a= T\g;    % a(1)= pos a(2)= vel   a(3)= acel
%primer punt0 

y= a(1)+a(2)*(t)+a(3)*(t.^2)+a(4)*(t.^3)+a(5)*(t.^4)+a(6)*(t.^5);
yd= a(2)+2*a(3)*(t)+3*a(4)*(t.^2)+4*a(5)*(t.^3)+5*a(6)*(t.^4);
ydd= 2*a(3)+6*a(4)*(t)+12*a(5)*(t.^2)+20*a(6)*(t.^3);

else
if (t>3)&&(t<=6)
    
    %% segundo punto 

t0=3; tf=6 
v0=0;  vf=0;
alpha0=0;  alphaf=0; 
q0=-2.69; qf=-2.6481; 



T=[1 t0  t0^2  t0^3   t0^4      t0^5;
   0  1 2*t0 3*t0^2 4*t0^3    5*t0^4;
   0  0   2   6*t0  12*t0^2   20*t0^3;
   1  tf  tf^2 tf^3  tf^4      tf^5;
   0  1   2*tf  3*tf^2  4*tf^3  5*tf^4;
   0  0   2      6*tf    12*tf^2  20*tf^3];


g=[q0;v0;alpha0;qf;vf;alphaf];
a=T\g;    % a(1)= pos a(2)= vel   a(3)= acel

y= a(1)+a(2)*(t)+a(3)*(t.^2)+a(4)*(t.^3)+a(5)*(t.^4)+a(6)*(t.^5);
yd= a(2)+2*a(3)*(t)+3*a(4)*(t.^2)+4*a(5)*(t.^3)+5*a(6)*(t.^4);
ydd= 2*a(3)+6*a(4)*(t)+12*a(5)*(t.^2)+20*a(6)*(t.^3);

else
 if (t>6)&&(t<=9)
%% tercer punto 
t0=6; tf=9;  
v0=0;  vf=0;
alpha0=0;   alphaf=0;
q0=-2.6481; qf=-2.58;   

%vf alphaf q0 para efectos practicos


T=[1 t0  t0^2  t0^3   t0^4      t0^5;
   0  1 2*t0 3*t0^2 4*t0^3    5*t0^4;
   0  0   2   6*t0  12*t0^2   20*t0^3;
   1  tf  tf^2 tf^3  tf^4      tf^5;
   0  1   2*tf  3*tf^2  4*tf^3  5*tf^4;
   0  0   2      6*tf    12*tf^2  20*tf^3];

g=[q0;v0;alpha0;qf;vf;alphaf];
a=T\g;    % a(1)= pos a(2)= vel   a(3)= acel
%primer puntp q=[0 10] donde q=[q0 qf]
y= a(1)+a(2)*(t)+a(3)*(t.^2)+a(4)*(t.^3)+a(5)*(t.^4)+a(6)*(t.^5);
yd= a(2)+2*a(3)*(t)+3*a(4)*(t.^2)+4*a(5)*(t.^3)+5*a(6)*(t.^4);
ydd= 2*a(3)+6*a(4)*(t)+12*a(5)*(t.^2)+20*a(6)*(t.^3);

else
 if (t>9)&&(t<=12)
%% cuarto punto 
t0=9; tf=12;  v0=0; alpha0=0; qf=-2.5498 ;  alphaf=0; q0=-2.58; vf=0;  


T=[1 t0  t0^2  t0^3   t0^4      t0^5;
   0  1 2*t0 3*t0^2 4*t0^3    5*t0^4;
   0  0   2   6*t0  12*t0^2   20*t0^3;
   1  tf  tf^2 tf^3  tf^4      tf^5;
   0  1   2*tf  3*tf^2  4*tf^3  5*tf^4;
   0  0   2      6*tf    12*tf^2  20*tf^3];


g=[q0;v0;alpha0;qf;vf;alphaf];
a=T\g;    % a(1)= pos a(2)= vel   a(3)= acel
%primer puntp q=[0 10] donde q=[q0 qf]

y= a(1)+a(2)*(t)+a(3)*(t.^2)+a(4)*(t.^3)+a(5)*(t.^4)+a(6)*(t.^5);
yd= a(2)+2*a(3)*(t)+3*a(4)*(t.^2)+4*a(5)*(t.^3)+5*a(6)*(t.^4);
ydd= 2*a(3)+6*a(4)*(t)+12*a(5)*(t.^2)+20*a(6)*(t.^3);

else
 if (t>12)&&(t<=15)
%% Quinto punto
     t0=12; tf=15;  v0=0; alpha0=0; qf=-2.80; alphaf=0; q0=-2.5498; vf=0;  


T=[1 t0  t0^2  t0^3   t0^4      t0^5;
   0  1 2*t0 3*t0^2 4*t0^3    5*t0^4;
   0  0   2   6*t0  12*t0^2   20*t0^3;
   1  tf  tf^2 tf^3  tf^4      tf^5;
   0  1   2*tf  3*tf^2  4*tf^3  5*tf^4;
   0  0   2      6*tf    12*tf^2  20*tf^3];

g=[q0;v0;alpha0;qf;vf;alphaf];
a=T\g;    % a(1)= pos a(2)= vel   a(3)= acel

y= a(1)+a(2)*(t)+a(3)*(t.^2)+a(4)*(t.^3)+a(5)*(t.^4)+a(6)*(t.^5);
yd= a(2)+2*a(3)*(t)+3*a(4)*(t.^2)+4*a(5)*(t.^3)+5*a(6)*(t.^4);
ydd= 2*a(3)+6*a(4)*(t)+12*a(5)*(t.^2)+20*a(6)*(t.^3);

else
      if t>15
           ydd=0;
           yd=0;
           y=0;
      end
end
end
end
end
end

== matlab function gtrackpol15/Control1 /MATLAB Function5 ==
  data: y output; t input; yd output; ydd output

function [y,yd,ydd] = qdd(t)
y=0;
yd=0;
ydd=0;
%a=[0 0 0 0 0 0]
if (t>0)&&(t<=3)
 
t0=0; tf=3; 
 v0=0; alpha0=0; qf=0.9828 ; 
 vf=0; alphaf=0; q0=0;  
%vf alphaf q0 para efectos practicos



T=[1 t0  t0^2  t0^3   t0^4      t0^5;
   0  1 2*t0 3*t0^2 4*t0^3    5*t0^4;
   0  0   2   6*t0  12*t0^2   20*t0^3;
   1  tf  tf^2 tf^3  tf^4      tf^5;
   0  1   2*tf  3*tf^2  4*tf^3  5*tf^4;
   0  0   2      6*tf    12*tf^2  20*tf^3];


g=[q0;v0;alpha0;qf;vf;alphaf];
a= T\g;    % a(1)= pos a(2)= vel   a(3)= acel
%primer punt0 

y= a(1)+a(2)*(t)+a(3)*(t.^2)+a(4)*(t.^3)+a(5)*(t.^4)+a(6)*(t.^5);
yd= a(2)+2*a(3)*(t)+3*a(4)*(t.^2)+4*a(5)*(t.^3)+5*a(6)*(t.^4);
ydd= 2*a(3)+6*a(4)*(t)+12*a(5)*(t.^2)+20*a(6)*(t.^3);

else
if (t>3)&&(t<=6)
    
    %% segundo punto 

t0=3; tf=6; 
v0=0;  vf=0;
alpha0=0;  alphaf=0; 
q0=0.9828; qf=0.9151 ; 



T=[1 t0  t0^2  t0^3   t0^4      t0^5;
   0  1 2*t0 3*t0^2 4*t0^3    5*t0^4;
   0  0   2   6*t0  12*t0^2   20*t0^3;
   1  tf  tf^2 tf^3  tf^4      tf^5;
   0  1   2*tf  3*tf^2  4*tf^3  5*tf^4;
   0  0   2      6*tf    12*tf^2  20*tf^3];


g=[q0;v0;alpha0;qf;vf;alphaf];
a=T\g;    % a(1)= pos a(2)= vel   a(3)= acel

y= a(1)+a(2)*(t)+a(3)*(t.^2)+a(4)*(t.^3)+a(5)*(t.^4)+a(6)*(t.^5);
yd= a(2)+2*a(3)*(t)+3*a(4)*(t.^2)+4*a(5)*(t.^3)+5*a(6)*(t.^4);
ydd= 2*a(3)+6*a(4)*(t)+12*a(5)*(t.^2)+20*a(6)*(t.^3);

else
 if (t>6)&&(t<=9)
%% tercer punto 
t0=6; tf=9;  
v0=0;  vf=0;
alpha0=0;   alphaf=0;
q0=0.9151; qf=0.8176 ;   

%vf alphaf q0 para efectos practicos


T=[1 t0  t0^2  t0^3   t0^4      t0^5;
   0  1 2*t0 3*t0^2 4*t0^3    5*t0^4;
   0  0   2   6*t0  12*t0^2   20*t0^3;
   1  tf  tf^2 tf^3  tf^4      tf^5;
   0  1   2*tf  3*tf^2  4*tf^3  5*tf^4;
   0  0   2      6*tf    12*tf^2  20*tf^3];

g=[q0;v0;alpha0;qf;vf;alphaf];
a=T\g;    % a(1)= pos a(2)= vel   a(3)= acel
%primer puntp q=[0 10] donde q=[q0 qf]
y= a(1)+a(2)*(t)+a(3)*(t.^2)+a(4)*(t.^3)+a(5)*(t.^4)+a(6)*(t.^5);
yd= a(2)+2*a(3)*(t)+3*a(4)*(t.^2)+4*a(5)*(t.^3)+5*a(6)*(t.^4);
ydd= 2*a(3)+6*a(4)*(t)+12*a(5)*(t.^2)+20*a(6)*(t.^3);

else
 if (t>9)&&(t<=12)
%% cuarto punto 
t0=9; tf=12;  v0=0; alpha0=0; qf=0.8157 ; alphaf=0; q0=0.8176; vf=0;  


T=[1 t0  t0^2  t0^3   t0^4      t0^5;
   0  1 2*t0 3*t0^2 4*t0^3    5*t0^4;
   0  0   2   6*t0  12*t0^2   20*t0^3;
   1  tf  tf^2 tf^3  tf^4      tf^5;
   0  1   2*tf  3*tf^2  4*tf^3  5*tf^4;
   0  0   2      6*tf    12*tf^2  20*tf^3];


g=[q0;v0;alpha0;qf;vf;alphaf];
a=T\g;    % a(1)= pos a(2)= vel   a(3)= acel
%primer puntp q=[0 10] donde q=[q0 qf]

y= a(1)+a(2)*(t)+a(3)*(t.^2)+a(4)*(t.^3)+a(5)*(t.^4)+a(6)*(t.^5);
yd= a(2)+2*a(3)*(t)+3*a(4)*(t.^2)+4*a(5)*(t.^3)+5*a(6)*(t.^4);
ydd= 2*a(3)+6*a(4)*(t)+12*a(5)*(t.^2)+20*a(6)*(t.^3);

else
 if (t>12)&&(t<=15)
     %% Quinto punto 

     t0=12; tf=15;  v0=0; alpha0=0; qf=0.9601 ; vf=0; alphaf=0; q0=0.8157; 


T=[1 t0  t0^2  t0^3   t0^4      t0^5;
   0  1 2*t0 3*t0^2 4*t0^3    5*t0^4;
   0  0   2   6*t0  12*t0^2   20*t0^3;
   1  tf  tf^2 tf^3  tf^4      tf^5;
   0  1   2*tf  3*tf^2  4*tf^3  5*tf^4;
   0  0   2      6*tf    12*tf^2  20*tf^3];

g=[q0;v0;alpha0;qf;vf;alphaf];
a=T\g;    % a(1)= pos a(2)= vel   a(3)= acel

y= a(1)+a(2)*(t)+a(3)*(t.^2)+a(4)*(t.^3)+a(5)*(t.^4)+a(6)*(t.^5);
yd= a(2)+2*a(3)*(t)+3*a(4)*(t.^2)+4*a(5)*(t.^3)+5*a(6)*(t.^4);
ydd= 2*a(3)+6*a(4)*(t)+12*a(5)*(t.^2)+20*a(6)*(t.^3);

else
      if t>15
           ydd=ydd;
           yd=yd;
           y=y;
      end
end
end
end
end
end
